simulink model "sh1"  (Simulink 6.6)
settings: Solver=ode45  StartTime=0.0  StopTime=10.0  RelTol=1e-3
libraries: cdsFilt x66, cdsEpicsIn x10, cdsWD x7, cdsMuxMatrix x4, cdsEpicsOut x2, cdsDio x2, dac x1, cdsEpicsBinIn x1, cdsParameters x1
(part 1 of 4)
settings Model: Creator=ligo  LastModifiedBy=ligo  ExtModeAutoUpdateStatusClock=off

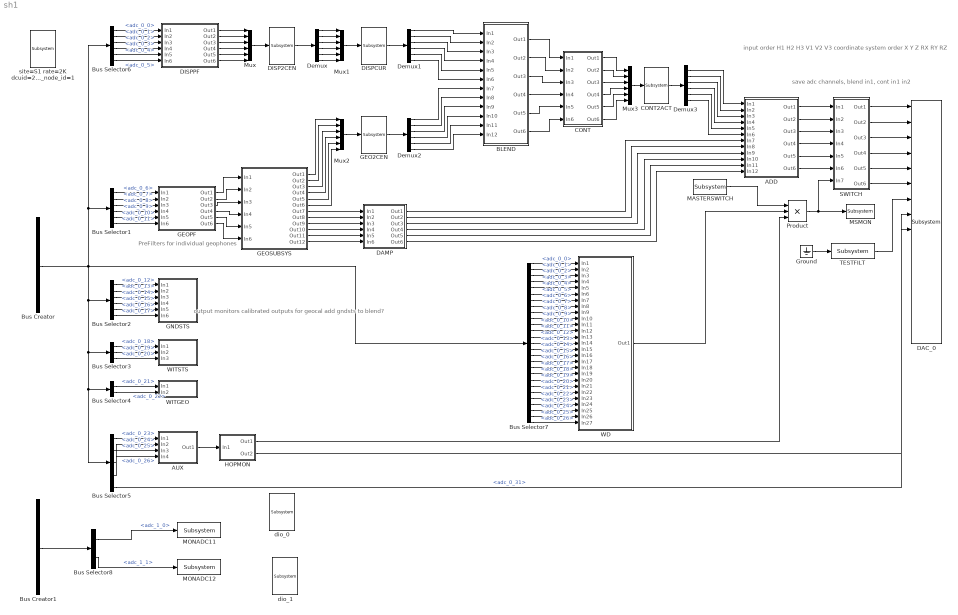
== system sh1 ==
  note: input order
      | H1 H2 H3 V1 V2 V3
      |
      | coordinate system order
      | X Y Z RX RY RZ
  note: save adc channels, blend in1, cont in1 in2
  note: PreFilters for
      | individual geophones
  note: output monitors
      |
      | calibrated outputs for geocal
      |
      | add gndsts to blend?
  ADD : Subsystem
  AUX : Subsystem
  BLEND : Subsystem
  Bus Creator : BusCreator  Tag=adc_0  Description=ADC0  Inputs='adc_0_0','adc_0_1','adc_0_2','adc_0_3','adc_0_4','adc_0_5','adc_0_6','adc_0_7','adc_0_8','adc_0_9','adc_0_10','adc_0_11','adc_0_12','adc_0_13','adc_0_14','adc_0_15','adc_0_16','adc_0_17','adc_0_18','adc_0_19','adc_0_20','adc_0_21','adc_0_22','adc_0_23','adc_0_24','adc_0_25','adc_0_26','adc_0_27','adc_0_28','adc_0_29','adc_0_30','adc_0_31'
      settings: AttributesFormatString=%<Tag>
  Bus Creator1 : BusCreator  Tag=adc_1  Description=ADC1  Inputs='adc_1_0','adc_1_1','adc_1_2','adc_1_3','adc_1_4','adc_1_5','adc_1_6','adc_1_7','adc_1_8','adc_1_9','adc_1_10','adc_1_11','adc_1_12','adc_1_13','adc_1_14','adc_1_15','adc_1_16','adc_1_17','adc_1_18','adc_1_19','adc_1_20','adc_1_21','adc_1_22','adc_1_23','adc_1_24','adc_1_25','adc_1_26','adc_1_27','adc_1_28','adc_1_29','adc_1_30','adc_1_31'
      settings: AttributesFormatString=%<Tag>
  Bus Selector1 : BusSelector  Description=ADC Selector  OutputSignals=adc_0_6,adc_0_7,adc_0_8,adc_0_9,adc_0_10,adc_0_11
      settings: AttributesFormatString=%<Description>
  Bus Selector2 : BusSelector  Description=ADC Selector  OutputSignals=adc_0_12,adc_0_13,adc_0_14,adc_0_15,adc_0_16,adc_0_17
      settings: AttributesFormatString=%<Description>
  Bus Selector3 : BusSelector  Description=ADC Selector  OutputSignals=adc_0_18,adc_0_19,adc_0_20
      settings: AttributesFormatString=%<Description>
  Bus Selector4 : BusSelector  Description=ADC Selector  OutputSignals=adc_0_21,adc_0_22
      settings: AttributesFormatString=%<Description>
  Bus Selector5 : BusSelector  Description=ADC Selector  OutputSignals=adc_0_23,adc_0_24,adc_0_25,adc_0_26,adc_0_31
      settings: AttributesFormatString=%<Description>
  Bus Selector6 : BusSelector  Description=ADC Selector  OutputSignals=adc_0_0,adc_0_1,adc_0_2,adc_0_3,adc_0_4,adc_0_5
      settings: AttributesFormatString=%<Description>
  Bus Selector7 : BusSelector  Description=ADC Selector  OutputSignals=adc_0_0,adc_0_1,adc_0_2,adc_0_3,adc_0_4,adc_0_5,adc_0_6,adc_0_7,adc_0_8,adc_0_9,adc_0_10,adc_0_11,adc_0_12,adc_0_13,adc_0_14,adc_0_15,adc_0_16,adc_0_17,adc_0_18,adc_0_19,adc_0_20,adc_0_21,adc_0_22,adc_0_23,adc_0_24,adc_0_25,adc_0_26
      settings: AttributesFormatString=%<Description>
  Bus Selector8 : BusSelector  Description=ADC Selector  OutputSignals=adc_1_0,adc_1_1
      settings: AttributesFormatString=%<Description>
  CONT : Subsystem
  CONT2ACT : cdsMuxMatrix/Subsystem  Tag=cdsMuxMatrix  Description=Any size matrix. Inputs and outputs must be connected using Mux and Demux parts.  SystemSampleTime=-1
      settings: AttributesFormatString=%<Tag>
  DAC_0 : dac/Subsystem  Description=DAC  SystemSampleTime=-1
      settings: AttributesFormatString=%<Description>
  DAMP : Subsystem
  DISP2CEN : cdsMuxMatrix/Subsystem  Tag=cdsMuxMatrix  Description=Any size matrix. Inputs and outputs must be connected using Mux and Demux parts.  SystemSampleTime=-1
      settings: AttributesFormatString=%<Tag>
  DISPCUR : cdsMuxMatrix/Subsystem  Tag=cdsMuxMatrix  Description=Any size matrix. Inputs and outputs must be connected using Mux and Demux parts.  SystemSampleTime=-1
      settings: AttributesFormatString=%<Tag>
  DISPPF : Subsystem
  Demux{,1..3} (4 alike) : Demux  Outputs=6
  GEO2CEN : cdsMuxMatrix/Subsystem  Tag=cdsMuxMatrix  Description=Any size matrix. Inputs and outputs must be connected using Mux and Demux parts.  SystemSampleTime=-1
      settings: AttributesFormatString=%<Tag>
  GEOPF : Subsystem
  GEOSUBSYS : Subsystem
  GNDSTS : Subsystem
  Ground : Ground
  HOPMON : Subsystem
  MASTERSWITCH : cdsEpicsBinIn/Subsystem  Tag=cdsEpicsBinIn  Description=|  SystemSampleTime=-1
      | Purpose:                                                                            
      | Create an EPICS binary (0 or 1) input channel to the FE realtime controls.          
      |                                                                                     
      | Operation:                                                                          
      | Outputs value from an EPICS ai record. Value is binary input (bi Epics record type).
      |                                                                                     
      | Usage:                                                                              
      | Name the part with the desired EPICS channel name.
      settings: AttributesFormatString=%<Tag>
  MONADC11 : cdsFilt/Subsystem  Tag=cdsFilt  Description=|  SystemSampleTime=-1
      | Purpose:                                                                                                                                                                                                                                  
      | Standard CDS IIR filter module.                                                                                                                                                                                                           
      |                                                                                                                                                                                                                                           
      | Operation:                                                                                                                                                                                                                                
      | Consists of 10 second order section IIR filters, plus a ramped gain stage. In FE code, also provides pre-defined test points and excitation channel inputs. The filter coefficients are defined in the LIGO system using the 'foton' tool.
      |                                                                                                                                                                                                                                           
      | Usage:                                                                                                                                                                                                                                    
      | Name the part with the desired filter module name.
      settings: AttributesFormatString=%<Tag>
  MONADC12 : cdsFilt/Subsystem  Tag=cdsFilt  Description=|  SystemSampleTime=-1
      | Purpose:                                                                                                                                                                                                                                  
      | Standard CDS IIR filter module.                                                                                                                                                                                                           
      |                                                                                                                                                                                                                                           
      | Operation:                                                                                                                                                                                                                                
      | Consists of 10 second order section IIR filters, plus a ramped gain stage. In FE code, also provides pre-defined test points and excitation channel inputs. The filter coefficients are defined in the LIGO system using the 'foton' tool.
      |                                                                                                                                                                                                                                           
      | Usage:                                                                                                                                                                                                                                    
      | Name the part with the desired filter module name.
      settings: AttributesFormatString=%<Tag>
  MSMON : cdsEpicsOut/Subsystem  Tag=cdsEpicsOutput  Description=|  SystemSampleTime=-1
      | Purpose:                                          
      | Output a FE signal to an EPICS channel.           
      |                                                   
      | Operation:                                        
      | Takes input value and passes it to EPICS record.  
      |                                                   
      | Usage:                                            
      | Name the part with the desired EPICS rrecord name.
      settings: AttributesFormatString=%<Tag>
  Mux{,1..3} (4 alike) : Mux  Inputs=6
  Product : Product  Inputs=3  RndMeth=Zero
  SWITCH : Subsystem
  TESTFILT : cdsFilt/Subsystem  Tag=cdsFilt  Description=|  SystemSampleTime=-1
      | Purpose:                                                                                                                                                                                                                                  
      | Standard CDS IIR filter module.                                                                                                                                                                                                           
      |                                                                                                                                                                                                                                           
      | Operation:                                                                                                                                                                                                                                
      | Consists of 10 second order section IIR filters, plus a ramped gain stage. In FE code, also provides pre-defined test points and excitation channel inputs. The filter coefficients are defined in the LIGO system using the 'foton' tool.
      |                                                                                                                                                                                                                                           
      | Usage:                                                                                                                                                                                                                                    
      | Name the part with the desired filter module name.
      settings: AttributesFormatString=%<Tag>
  WD : Subsystem
  WITGEO : Subsystem
  WITSTS : Subsystem
  dio_0 : cdsDio/Subsystem  Description=|  SystemSampleTime=-1
      | support for 8 bit input 8 bit output DIO PCI card
      | ACCESS I/O Products model DIO-24D
  dio_1 : cdsDio/Subsystem  Description=|  SystemSampleTime=-1
      | support for 8 bit input 8 bit output DIO PCI card
      | ACCESS I/O Products model DIO-24D
  site=S1 rate=2K dcuid=22 gds_node_id=1 : cdsParameters/Subsystem  Tag=cdsParameters  SystemSampleTime=-1
      settings: AttributesFormatString=%<Tag>
  wires:
  Bus Creator/1 -> Bus Selector2/1, Bus Selector3/1, Bus Selector4/1, Bus Selector5/1, Bus Selector6/1, Bus Selector1/1, Bus Selector7/1
  Mux/1 -> DISP2CEN/1
  DISP2CEN/1 -> Demux/1
  Mux1/1 -> DISPCUR/1
  DISPCUR/1 -> Demux1/1
  Demux/1 -> Mux1/1
  Demux/2 -> Mux1/2
  Demux/3 -> Mux1/3
  Demux/4 -> Mux1/4
  Demux/5 -> Mux1/5
  Demux/6 -> Mux1/6
  Mux2/1 -> GEO2CEN/1
  GEO2CEN/1 -> Demux2/1
  Mux3/1 -> CONT2ACT/1
  CONT2ACT/1 -> Demux3/1
  Bus Selector1/1 -> GEOPF/1(In1)  "<adc_0_6>"
  Bus Selector1/2 -> GEOPF/2(In2)  "<adc_0_7>"
  Bus Selector1/3 -> GEOPF/3(In3)  "<adc_0_8>"
  Bus Selector1/4 -> GEOPF/4(In4)  "<adc_0_9>"
  Bus Selector1/5 -> GEOPF/5(In5)  "<adc_0_10>"
  Bus Selector1/6 -> GEOPF/6(In6)  "<adc_0_11>"
  Bus Selector2/1 -> GNDSTS/1(In1)  "<adc_0_12>"
  Bus Selector2/2 -> GNDSTS/2(In2)  "<adc_0_13>"
  Bus Selector2/3 -> GNDSTS/3(In3)  "<adc_0_14>"
  Bus Selector2/4 -> GNDSTS/4(In4)  "<adc_0_15>"
  Bus Selector2/5 -> GNDSTS/5(In5)  "<adc_0_16>"
  Bus Selector2/6 -> GNDSTS/6(In6)  "<adc_0_17>"
  Bus Selector3/1 -> WITSTS/1(In1)  "<adc_0_18>"
  Bus Selector3/2 -> WITSTS/2(In2)  "<adc_0_19>"
  Bus Selector3/3 -> WITSTS/3(In3)  "<adc_0_20>"
  Bus Selector4/1 -> WITGEO/1(In1)  "<adc_0_21>"
  Bus Selector4/2 -> WITGEO/2(In2)  "<adc_0_22>"
  Bus Selector5/1 -> AUX/1(In1)  "<adc_0_23>"
  Bus Selector5/2 -> AUX/2(In2)  "<adc_0_24>"
  Bus Selector5/3 -> AUX/3(In3)  "<adc_0_25>"
  Bus Selector5/4 -> AUX/4(In4)  "<adc_0_26>"
  Bus Selector6/1 -> DISPPF/1(In1)  "<adc_0_0>"
  Bus Selector6/2 -> DISPPF/2(In2)  "<adc_0_1>"
  Bus Selector6/3 -> DISPPF/3(In3)  "<adc_0_2>"
  Bus Selector6/4 -> DISPPF/4(In4)  "<adc_0_3>"
  Bus Selector6/5 -> DISPPF/5(In5)  "<adc_0_4>"
  Bus Selector6/6 -> DISPPF/6(In6)  "<adc_0_5>"
  DISPPF/1(Out1) -> Mux/1
  DISPPF/2(Out2) -> Mux/2
  DISPPF/3(Out3) -> Mux/3
  DISPPF/4(Out4) -> Mux/4
  DISPPF/5(Out5) -> Mux/5
  DISPPF/6(Out6) -> Mux/6
  DAMP/1(Out1) -> ADD/7(In7)
  DAMP/2(Out2) -> ADD/8(In8)
  DAMP/3(Out3) -> ADD/9(In9)
  DAMP/4(Out4) -> ADD/10(In10)
  DAMP/5(Out5) -> ADD/11(In11)
  DAMP/6(Out6) -> ADD/12(In12)
  Demux3/1 -> ADD/1(In1)
  Demux3/2 -> ADD/2(In2)
  Demux3/3 -> ADD/3(In3)
  Demux3/4 -> ADD/4(In4)
  Demux3/5 -> ADD/5(In5)
  Demux3/6 -> ADD/6(In6)
  ADD/1(Out1) -> SWITCH/1(In1)
  ADD/2(Out2) -> SWITCH/2(In2)
  ADD/3(Out3) -> SWITCH/3(In3)
  ADD/4(Out4) -> SWITCH/4(In4)
  ADD/5(Out5) -> SWITCH/5(In5)
  ADD/6(Out6) -> SWITCH/6(In6)
  SWITCH/1(Out1) -> DAC_0/1
  SWITCH/2(Out2) -> DAC_0/2
  SWITCH/3(Out3) -> DAC_0/3
  SWITCH/4(Out4) -> DAC_0/4
  SWITCH/5(Out5) -> DAC_0/5
  SWITCH/6(Out6) -> DAC_0/6
  GEOPF/1(Out1) -> GEOSUBSYS/1(In1)
  GEOPF/2(Out2) -> GEOSUBSYS/2(In2)
  GEOPF/3(Out3) -> GEOSUBSYS/3(In3)
  GEOPF/4(Out4) -> GEOSUBSYS/4(In4)
  GEOPF/5(Out5) -> GEOSUBSYS/5(In5)
  GEOPF/6(Out6) -> GEOSUBSYS/6(In6)
  GEOSUBSYS/1(Out1) -> Mux2/1
  GEOSUBSYS/2(Out2) -> Mux2/2
  GEOSUBSYS/3(Out3) -> Mux2/3
  GEOSUBSYS/4(Out4) -> Mux2/4
  GEOSUBSYS/5(Out5) -> Mux2/5
  GEOSUBSYS/6(Out6) -> Mux2/6
  GEOSUBSYS/7(Out7) -> DAMP/1(In1)
  GEOSUBSYS/8(Out8) -> DAMP/2(In2)
  GEOSUBSYS/9(Out9) -> DAMP/3(In3)
  GEOSUBSYS/10(Out10) -> DAMP/4(In4)
  GEOSUBSYS/11(Out11) -> DAMP/5(In5)
  GEOSUBSYS/12(Out12) -> DAMP/6(In6)
  Demux1/1 -> BLEND/1(In1)
  Demux1/2 -> BLEND/2(In2)
  Demux1/3 -> BLEND/3(In3)
  Demux1/4 -> BLEND/4(In4)
  Demux1/5 -> BLEND/5(In5)
  Demux1/6 -> BLEND/6(In6)
  Demux2/1 -> BLEND/7(In7)
  Demux2/2 -> BLEND/8(In8)
  Demux2/3 -> BLEND/9(In9)
  Demux2/4 -> BLEND/10(In10)
  Demux2/5 -> BLEND/11(In11)
  Demux2/6 -> BLEND/12(In12)
  BLEND/1(Out1) -> CONT/1(In1)
  BLEND/2(Out2) -> CONT/2(In2)
  BLEND/3(Out3) -> CONT/3(In3)
  BLEND/4(Out4) -> CONT/4(In4)
  BLEND/5(Out5) -> CONT/5(In5)
  BLEND/6(Out6) -> CONT/6(In6)
  CONT/1(Out1) -> Mux3/1
  CONT/2(Out2) -> Mux3/2
  CONT/3(Out3) -> Mux3/3
  CONT/4(Out4) -> Mux3/4
  CONT/5(Out5) -> Mux3/5
  CONT/6(Out6) -> Mux3/6
  Product/1 -> MSMON/1, SWITCH/7(In7)
  MASTERSWITCH/1 -> Product/1
  TESTFILT/1 -> DAC_0/7
  AUX/1(Out1) -> HOPMON/1(In1)
  Bus Selector7/1 -> WD/1(In1)  "<adc_0_0>"
  Bus Selector7/2 -> WD/2(In2)  "<adc_0_1>"
  Bus Selector7/3 -> WD/3(In3)  "<adc_0_2>"
  Bus Selector7/4 -> WD/4(In4)  "<adc_0_3>"
  Bus Selector7/5 -> WD/5(In5)  "<adc_0_4>"
  Bus Selector7/6 -> WD/6(In6)  "<adc_0_5>"
  Bus Selector7/7 -> WD/7(In7)  "<adc_0_6>"
  Bus Selector7/8 -> WD/8(In8)  "<adc_0_7>"
  Bus Selector7/9 -> WD/9(In9)  "<adc_0_8>"
  Bus Selector7/10 -> WD/10(In10)  "<adc_0_9>"
  Bus Selector7/11 -> WD/11(In11)  "<adc_0_10>"
  Bus Selector7/12 -> WD/12(In12)  "<adc_0_11>"
  Bus Selector7/13 -> WD/13(In13)  "<adc_0_12>"
  Bus Selector7/14 -> WD/14(In14)  "<adc_0_13>"
  Bus Selector7/15 -> WD/15(In15)  "<adc_0_14>"
  Bus Selector7/16 -> WD/16(In16)  "<adc_0_15>"
  Bus Selector7/17 -> WD/17(In17)  "<adc_0_16>"
  Bus Selector7/18 -> WD/18(In18)  "<adc_0_17>"
  Bus Selector7/19 -> WD/19(In19)  "<adc_0_18>"
  Bus Selector7/20 -> WD/20(In20)  "<adc_0_19>"
  Bus Selector7/21 -> WD/21(In21)  "<adc_0_20>"
  Bus Selector7/22 -> WD/22(In22)  "<adc_0_21>"
  Bus Selector7/23 -> WD/23(In23)  "<adc_0_22>"
  Bus Selector7/24 -> WD/24(In24)  "<adc_0_23>"
  Bus Selector7/25 -> WD/25(In25)  "<adc_0_24>"
  Bus Selector7/26 -> WD/26(In26)  "<adc_0_25>"
  Bus Selector7/27 -> WD/27(In27)  "<adc_0_26>"
  WD/1(Out1) -> Product/2
  HOPMON/1(Out1) -> Product/3
  HOPMON/2(Out2) -> DAC_0/8
  Ground/1 -> TESTFILT/1
  Bus Creator1/1 -> Bus Selector8/1
  Bus Selector8/1 -> MONADC11/1  "<adc_1_0>"
  Bus Selector8/2 -> MONADC12/1  "<adc_1_1>"
  Bus Selector5/5 -> DAC_0/9  "<adc_0_31>"

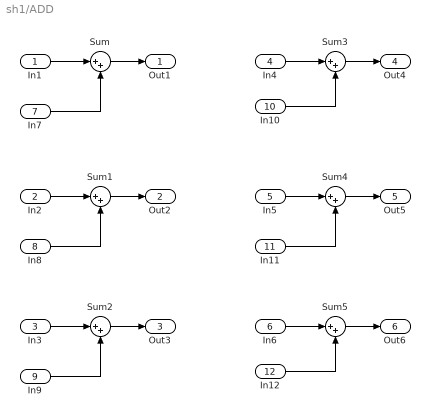
== system sh1/ADD ==
  In1 : Inport
  In2 : Inport  Port=2
  In3 : Inport  Port=3
  In4 : Inport  Port=4
  In5 : Inport  Port=5
  In6 : Inport  Port=6
  In7 : Inport  Port=7
  In8 : Inport  Port=8
  In9 : Inport  Port=9
  In10 : Inport  Port=10
  In11 : Inport  Port=11
  In12 : Inport  Port=12
  Sum{,1..5} (6 alike) : Sum  Inputs=|++
  Out1 : Outport
  Out2 : Outport  Port=2
  Out3 : Outport  Port=3
  Out4 : Outport  Port=4
  Out5 : Outport  Port=5
  Out6 : Outport  Port=6
  wires:
  Sum/1 -> Out1/1
  Sum1/1 -> Out2/1
  Sum2/1 -> Out3/1
  Sum3/1 -> Out4/1
  Sum4/1 -> Out5/1
  Sum5/1 -> Out6/1
  In1/1 -> Sum/1
  In2/1 -> Sum1/1
  In3/1 -> Sum2/1
  In4/1 -> Sum3/1
  In5/1 -> Sum4/1
  In6/1 -> Sum5/1
  In7/1 -> Sum/2
  In8/1 -> Sum1/2
  In9/1 -> Sum2/2
  In10/1 -> Sum3/2
  In11/1 -> Sum4/2
  In12/1 -> Sum5/2

== system sh1/AUX ==
  In1 : Inport
  In2 : Inport  Port=2
  In3 : Inport  Port=3
  In4 : Inport  Port=4
  A : cdsFilt/Subsystem  Tag=cdsFilt  Description=|  SystemSampleTime=-1
      | Purpose:                                                                                                                                                                                                                                  
      | Standard CDS IIR filter module.                                                                                                                                                                                                           
      |                                                                                                                                                                                                                                           
      | Operation:                                                                                                                                                                                                                                
      | Consists of 10 second order section IIR filters, plus a ramped gain stage. In FE code, also provides pre-defined test points and excitation channel inputs. The filter coefficients are defined in the LIGO system using the 'foton' tool.
      |                                                                                                                                                                                                                                           
      | Usage:                                                                                                                                                                                                                                    
      | Name the part with the desired filter module name.
      settings: AttributesFormatString=%<Tag>
  B : cdsFilt/Subsystem  Tag=cdsFilt  Description=|  SystemSampleTime=-1
      | Purpose:                                                                                                                                                                                                                                  
      | Standard CDS IIR filter module.                                                                                                                                                                                                           
      |                                                                                                                                                                                                                                           
      | Operation:                                                                                                                                                                                                                                
      | Consists of 10 second order section IIR filters, plus a ramped gain stage. In FE code, also provides pre-defined test points and excitation channel inputs. The filter coefficients are defined in the LIGO system using the 'foton' tool.
      |                                                                                                                                                                                                                                           
      | Usage:                                                                                                                                                                                                                                    
      | Name the part with the desired filter module name.
      settings: AttributesFormatString=%<Tag>
  C : cdsFilt/Subsystem  Tag=cdsFilt  Description=|  SystemSampleTime=-1
      | Purpose:                                                                                                                                                                                                                                  
      | Standard CDS IIR filter module.                                                                                                                                                                                                           
      |                                                                                                                                                                                                                                           
      | Operation:                                                                                                                                                                                                                                
      | Consists of 10 second order section IIR filters, plus a ramped gain stage. In FE code, also provides pre-defined test points and excitation channel inputs. The filter coefficients are defined in the LIGO system using the 'foton' tool.
      |                                                                                                                                                                                                                                           
      | Usage:                                                                                                                                                                                                                                    
      | Name the part with the desired filter module name.
      settings: AttributesFormatString=%<Tag>
  D : cdsFilt/Subsystem  Tag=cdsFilt  Description=|  SystemSampleTime=-1
      | Purpose:                                                                                                                                                                                                                                  
      | Standard CDS IIR filter module.                                                                                                                                                                                                           
      |                                                                                                                                                                                                                                           
      | Operation:                                                                                                                                                                                                                                
      | Consists of 10 second order section IIR filters, plus a ramped gain stage. In FE code, also provides pre-defined test points and excitation channel inputs. The filter coefficients are defined in the LIGO system using the 'foton' tool.
      |                                                                                                                                                                                                                                           
      | Usage:                                                                                                                                                                                                                                    
      | Name the part with the desired filter module name.
      settings: AttributesFormatString=%<Tag>
  Terminator : Terminator
  Terminator1 : Terminator
  Terminator2 : Terminator
  Out1 : Outport
  wires:
  In1/1 -> A/1
  In2/1 -> B/1
  B/1 -> Terminator1/1
  A/1 -> Terminator/1
  In3/1 -> C/1
  In4/1 -> D/1
  D/1 -> Out1/1
  C/1 -> Terminator2/1

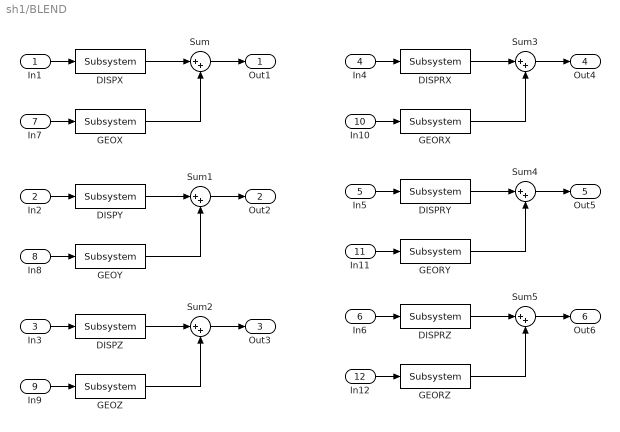
== system sh1/BLEND ==
  In1 : Inport
  In2 : Inport  Port=2
  In3 : Inport  Port=3
  In4 : Inport  Port=4
  In5 : Inport  Port=5
  In6 : Inport  Port=6
  In7 : Inport  Port=7
  In8 : Inport  Port=8
  In9 : Inport  Port=9
  In10 : Inport  Port=10
  In11 : Inport  Port=11
  In12 : Inport  Port=12
  DISPRX : cdsFilt/Subsystem  Tag=cdsFilt  Description=|  SystemSampleTime=-1
      | Purpose:                                                                                                                                                                                                                                  
      | Standard CDS IIR filter module.                                                                                                                                                                                                           
      |                                                                                                                                                                                                                                           
      | Operation:                                                                                                                                                                                                                                
      | Consists of 10 second order section IIR filters, plus a ramped gain stage. In FE code, also provides pre-defined test points and excitation channel inputs. The filter coefficients are defined in the LIGO system using the 'foton' tool.
      |                                                                                                                                                                                                                                           
      | Usage:                                                                                                                                                                                                                                    
      | Name the part with the desired filter module name.
      settings: AttributesFormatString=%<Tag>
  DISPRY : cdsFilt/Subsystem  Tag=cdsFilt  Description=|  SystemSampleTime=-1
      | Purpose:                                                                                                                                                                                                                                  
      | Standard CDS IIR filter module.                                                                                                                                                                                                           
      |                                                                                                                                                                                                                                           
      | Operation:                                                                                                                                                                                                                                
      | Consists of 10 second order section IIR filters, plus a ramped gain stage. In FE code, also provides pre-defined test points and excitation channel inputs. The filter coefficients are defined in the LIGO system using the 'foton' tool.
      |                                                                                                                                                                                                                                           
      | Usage:                                                                                                                                                                                                                                    
      | Name the part with the desired filter module name.
      settings: AttributesFormatString=%<Tag>
  DISPRZ : cdsFilt/Subsystem  Tag=cdsFilt  Description=|  SystemSampleTime=-1
      | Purpose:                                                                                                                                                                                                                                  
      | Standard CDS IIR filter module.                                                                                                                                                                                                           
      |                                                                                                                                                                                                                                           
      | Operation:                                                                                                                                                                                                                                
      | Consists of 10 second order section IIR filters, plus a ramped gain stage. In FE code, also provides pre-defined test points and excitation channel inputs. The filter coefficients are defined in the LIGO system using the 'foton' tool.
      |                                                                                                                                                                                                                                           
      | Usage:                                                                                                                                                                                                                                    
      | Name the part with the desired filter module name.
      settings: AttributesFormatString=%<Tag>
  DISPX : cdsFilt/Subsystem  Tag=cdsFilt  Description=|  SystemSampleTime=-1
      | Purpose:                                                                                                                                                                                                                                  
      | Standard CDS IIR filter module.                                                                                                                                                                                                           
      |                                                                                                                                                                                                                                           
      | Operation:                                                                                                                                                                                                                                
      | Consists of 10 second order section IIR filters, plus a ramped gain stage. In FE code, also provides pre-defined test points and excitation channel inputs. The filter coefficients are defined in the LIGO system using the 'foton' tool.
      |                                                                                                                                                                                                                                           
      | Usage:                                                                                                                                                                                                                                    
      | Name the part with the desired filter module name.
      settings: AttributesFormatString=%<Tag>
  DISPY : cdsFilt/Subsystem  Tag=cdsFilt  Description=|  SystemSampleTime=-1
      | Purpose:                                                                                                                                                                                                                                  
      | Standard CDS IIR filter module.                                                                                                                                                                                                           
      |                                                                                                                                                                                                                                           
      | Operation:                                                                                                                                                                                                                                
      | Consists of 10 second order section IIR filters, plus a ramped gain stage. In FE code, also provides pre-defined test points and excitation channel inputs. The filter coefficients are defined in the LIGO system using the 'foton' tool.
      |                                                                                                                                                                                                                                           
      | Usage:                                                                                                                                                                                                                                    
      | Name the part with the desired filter module name.
      settings: AttributesFormatString=%<Tag>
  DISPZ : cdsFilt/Subsystem  Tag=cdsFilt  Description=|  SystemSampleTime=-1
      | Purpose:                                                                                                                                                                                                                                  
      | Standard CDS IIR filter module.                                                                                                                                                                                                           
      |                                                                                                                                                                                                                                           
      | Operation:                                                                                                                                                                                                                                
      | Consists of 10 second order section IIR filters, plus a ramped gain stage. In FE code, also provides pre-defined test points and excitation channel inputs. The filter coefficients are defined in the LIGO system using the 'foton' tool.
      |                                                                                                                                                                                                                                           
      | Usage:                                                                                                                                                                                                                                    
      | Name the part with the desired filter module name.
      settings: AttributesFormatString=%<Tag>
  GEORX : cdsFilt/Subsystem  Tag=cdsFilt  Description=|  SystemSampleTime=-1
      | Purpose:                                                                                                                                                                                                                                  
      | Standard CDS IIR filter module.                                                                                                                                                                                                           
      |                                                                                                                                                                                                                                           
      | Operation:                                                                                                                                                                                                                                
      | Consists of 10 second order section IIR filters, plus a ramped gain stage. In FE code, also provides pre-defined test points and excitation channel inputs. The filter coefficients are defined in the LIGO system using the 'foton' tool.
      |                                                                                                                                                                                                                                           
      | Usage:                                                                                                                                                                                                                                    
      | Name the part with the desired filter module name.
      settings: AttributesFormatString=%<Tag>
  GEORY : cdsFilt/Subsystem  Tag=cdsFilt  Description=|  SystemSampleTime=-1
      | Purpose:                                                                                                                                                                                                                                  
      | Standard CDS IIR filter module.                                                                                                                                                                                                           
      |                                                                                                                                                                                                                                           
      | Operation:                                                                                                                                                                                                                                
      | Consists of 10 second order section IIR filters, plus a ramped gain stage. In FE code, also provides pre-defined test points and excitation channel inputs. The filter coefficients are defined in the LIGO system using the 'foton' tool.
      |                                                                                                                                                                                                                                           
      | Usage:                                                                                                                                                                                                                                    
      | Name the part with the desired filter module name.
      settings: AttributesFormatString=%<Tag>
  GEORZ : cdsFilt/Subsystem  Tag=cdsFilt  Description=|  SystemSampleTime=-1
      | Purpose:                                                                                                                                                                                                                                  
      | Standard CDS IIR filter module.                                                                                                                                                                                                           
      |                                                                                                                                                                                                                                           
      | Operation:                                                                                                                                                                                                                                
      | Consists of 10 second order section IIR filters, plus a ramped gain stage. In FE code, also provides pre-defined test points and excitation channel inputs. The filter coefficients are defined in the LIGO system using the 'foton' tool.
      |                                                                                                                                                                                                                                           
      | Usage:                                                                                                                                                                                                                                    
      | Name the part with the desired filter module name.
      settings: AttributesFormatString=%<Tag>
  GEOX : cdsFilt/Subsystem  Tag=cdsFilt  Description=|  SystemSampleTime=-1
      | Purpose:                                                                                                                                                                                                                                  
      | Standard CDS IIR filter module.                                                                                                                                                                                                           
      |                                                                                                                                                                                                                                           
      | Operation:                                                                                                                                                                                                                                
      | Consists of 10 second order section IIR filters, plus a ramped gain stage. In FE code, also provides pre-defined test points and excitation channel inputs. The filter coefficients are defined in the LIGO system using the 'foton' tool.
      |                                                                                                                                                                                                                                           
      | Usage:                                                                                                                                                                                                                                    
      | Name the part with the desired filter module name.
      settings: AttributesFormatString=%<Tag>
  GEOY : cdsFilt/Subsystem  Tag=cdsFilt  Description=|  SystemSampleTime=-1
      | Purpose:                                                                                                                                                                                                                                  
      | Standard CDS IIR filter module.                                                                                                                                                                                                           
      |                                                                                                                                                                                                                                           
      | Operation:                                                                                                                                                                                                                                
      | Consists of 10 second order section IIR filters, plus a ramped gain stage. In FE code, also provides pre-defined test points and excitation channel inputs. The filter coefficients are defined in the LIGO system using the 'foton' tool.
      |                                                                                                                                                                                                                                           
      | Usage:                                                                                                                                                                                                                                    
      | Name the part with the desired filter module name.
      settings: AttributesFormatString=%<Tag>
  GEOZ : cdsFilt/Subsystem  Tag=cdsFilt  Description=|  SystemSampleTime=-1
      | Purpose:                                                                                                                                                                                                                                  
      | Standard CDS IIR filter module.                                                                                                                                                                                                           
      |                                                                                                                                                                                                                                           
      | Operation:                                                                                                                                                                                                                                
      | Consists of 10 second order section IIR filters, plus a ramped gain stage. In FE code, also provides pre-defined test points and excitation channel inputs. The filter coefficients are defined in the LIGO system using the 'foton' tool.
      |                                                                                                                                                                                                                                           
      | Usage:                                                                                                                                                                                                                                    
      | Name the part with the desired filter module name.
      settings: AttributesFormatString=%<Tag>
  Sum{,1..5} (6 alike) : Sum  Inputs=|++
  Out1 : Outport
  Out2 : Outport  Port=2
  Out3 : Outport  Port=3
  Out4 : Outport  Port=4
  Out5 : Outport  Port=5
  Out6 : Outport  Port=6
  wires:
  In1/1 -> DISPX/1
  In7/1 -> GEOX/1
  DISPX/1 -> Sum/1
  GEOX/1 -> Sum/2
  Sum/1 -> Out1/1
  In2/1 -> DISPY/1
  In8/1 -> GEOY/1
  DISPY/1 -> Sum1/1
  GEOY/1 -> Sum1/2
  Sum1/1 -> Out2/1
  In3/1 -> DISPZ/1
  In9/1 -> GEOZ/1
  DISPZ/1 -> Sum2/1
  GEOZ/1 -> Sum2/2
  Sum2/1 -> Out3/1
  In4/1 -> DISPRX/1
  In10/1 -> GEORX/1
  DISPRX/1 -> Sum3/1
  GEORX/1 -> Sum3/2
  Sum3/1 -> Out4/1
  In5/1 -> DISPRY/1
  In11/1 -> GEORY/1
  DISPRY/1 -> Sum4/1
  GEORY/1 -> Sum4/2
  Sum4/1 -> Out5/1
  In6/1 -> DISPRZ/1
  In12/1 -> GEORZ/1
  DISPRZ/1 -> Sum5/1
  GEORZ/1 -> Sum5/2
  Sum5/1 -> Out6/1
